simulink model "VTOLDynamics"  (R2024b)
settings: Solver=ode23t  StartTime=0.0  StopTime=10.0  FixedStep=0.001  RelTol=1e-3
undefined symbols (not defined in the file): const, contact, env, F, Flap_Activate, iniRoll, initPitch, iniYaw, Light, Limit, MIL, motorctrl, tiltIni, uavParam, uavParams, vIni, xGround, yGround, zGround
libraries: matrix_library x8, slpidlib x4, robotcorelib x4, aerolibasang x2, aerolibwind2 x2, sharedtransform x2, shared6dof x1, aerolibadyn x1, sharedutil x1, Uav_Electrical_lib x1, aerolibatmos2 x1
(part 2 of 3)

== system VTOLDynamics/Force and Moments/Propulsion/Rotor1 Drag Torque ==
  note: RPM_2_rad/s
  note: Drage Torque Calculate
      |
      | Vertical takeoff :
      |
      | Q = rho * A * (Omega*R)^2 * R * CQ, where the unit of Q is [N-m]
  note: Parameters
      | rho : air density
      | A : rotor blade area
      | Omega : motor speed (rad/s)
      | CQ: motor torque coefficient
      | R : rotor blade radius
  Actuator : Inport
  Gain1 : Gain  Gain=uavParams.aero.air_density*uavParams.geom.RotorArea*(uavParams.geom.PropDiameter/2)^3*uavParams.rotor.Cq
  Gain8 : Gain  Gain=2*pi/60
  Square : Math  Operator=square
  Unit Delay : UnitDelay  SampleTime=0.001  HasFrameUpgradeWarning=on
  Out1 : Outport
  wires:
  Gain8/1 -> Square/1
  Square/1 -> Gain1/1
  Actuator/1 -> Gain8/1
  Gain1/1 -> Unit Delay/1
  Unit Delay/1 -> Out1/1

== system VTOLDynamics/Force and Moments/Propulsion/Rotor2 Drag Torque ==
  note: RPM_2_rad/s
  note: Drage Torque Calculate
  Actuator : Inport
  Gain1 : Gain  Gain=uavParams.aero.air_density*uavParams.geom.RotorArea*(uavParams.geom.PropDiameter/2)^3*uavParams.rotor.Cq
  Gain8 : Gain  Gain=2*pi/60
  Square : Math  Operator=square
  Unit Delay : UnitDelay  SampleTime=0.001  HasFrameUpgradeWarning=on
  Out2 : Outport
  wires:
  Gain8/1 -> Square/1
  Square/1 -> Gain1/1
  Actuator/1 -> Gain8/1
  Gain1/1 -> Unit Delay/1
  Unit Delay/1 -> Out2/1

== system VTOLDynamics/Force and Moments/Propulsion/Rotor3 Drag Torque ==
  note: RPM_2_rad/s
  note: Drage Torque Calculate
  Actuator : Inport
  Gain1 : Gain  Gain=uavParams.aero.air_density*uavParams.geom.RotorArea*(uavParams.geom.PropDiameter/2)^3*uavParams.rotor.Cq
  Gain8 : Gain  Gain=2*pi/60
  Square : Math  Operator=square
  Unit Delay : UnitDelay  SampleTime=0.001  HasFrameUpgradeWarning=on
  Out2 : Outport
  wires:
  Gain8/1 -> Square/1
  Square/1 -> Gain1/1
  Actuator/1 -> Gain8/1
  Gain1/1 -> Unit Delay/1
  Unit Delay/1 -> Out2/1

== system VTOLDynamics/Force and Moments/Propulsion/Rotor4 Drag Torque ==
  note: RPM_2_rad/s
  note: Drage Torque Calculate
  Actuator : Inport
  Gain1 : Gain  Gain=uavParams.aero.air_density*uavParams.geom.RotorArea*(uavParams.geom.PropDiameter/2)^3*uavParams.rotor.Cq
  Gain8 : Gain  Gain=2*pi/60
  Square : Math  Operator=square
  Unit Delay : UnitDelay  SampleTime=0.001  HasFrameUpgradeWarning=on
  Out1 : Outport
  wires:
  Gain8/1 -> Square/1
  Square/1 -> Gain1/1
  Actuator/1 -> Gain8/1
  Gain1/1 -> Unit Delay/1
  Unit Delay/1 -> Out1/1

== system VTOLDynamics/Force and Moments/Propulsion/Tilt Servo Dynamics ==
  TiltA : Inport
  TiltB : Inport  Port=2
  Gain2 : Gain  Gain=pi/2
  Gain3 : Gain  Gain=pi/2
  IC : InitialCondition  Value=tiltIni
  IC1 : InitialCondition  Value=tiltIni
  Servo Dynamics : TransferFcn  Numerator=uavParams.tiltservo.tfnum  Denominator=uavParams.tiltservo.tfden
  Servo Dynamics1 : TransferFcn  Numerator=uavParams.tiltservo.tfnum  Denominator=uavParams.tiltservo.tfden
  Tilt1 : Outport
  Tilt2 : Outport  Port=2
  wires:
  Gain2/1 -> Servo Dynamics/1
  TiltB/1 -> Gain3/1
  Servo Dynamics/1 -> IC1/1
  Servo Dynamics1/1 -> IC/1
  IC/1 -> Tilt2/1  "Tilt2"
  IC1/1 -> Tilt1/1  "Tilt1"
  Gain3/1 -> Servo Dynamics1/1
  TiltA/1 -> Gain2/1

== system VTOLDynamics/Force and Moments/Weather Model/Simple Model ==
  note: #11, 25/07/04, MH, Fixed
      | Use International Standard Atmosphere model
      | to obtain the air density varying with altitude
  AirData : Inport
  Xe : Inport  Port=2
  Euler : Inport  Port=3
  Constant : Constant  Value=[ 0 0 0]
      settings: AttributesFormatString=%<Value>
  Constant1 : Constant  Commented=on  Value=const.rho0
  Gain : Gain  Gain=-1
  ISA Atmosphere Model : aerolibatmos2/ISA Atmosphere Model  useExtended=off  action=Warning  custom=off  viscosityOut=off  g=9.80665  gamma=1.4  R=287.0531  L=0.0065  h_trop=11000  h_strat=20000  rho0=1.225  P0=101325  T0=288.15  h0=0  S=110.4  Tref=273.15  muref=1.716e-5
  Selector : Selector  InputPortWidth=3  IndexOptions=Index vector (dialog)  Indices=[3]  OutputSizes=1
  Terminator{,1..4} (5 alike) : Terminator
  Wind_e : Outport  Unit=m/s  VectorParamsAs1DForOutWhenUnconnected=off
  " Rho" : Outport  Port=2  VectorParamsAs1DForOutWhenUnconnected=off
  wires:
  AirData/1 -> Terminator/1
  Constant/1 -> Wind_e/1
  Euler/1 -> Terminator1/1
  Xe/1 -> Selector/1
  Selector/1 -> Gain/1
  Gain/1 -> ISA Atmosphere Model/1
  ISA Atmosphere Model/1 -> Terminator2/1
  ISA Atmosphere Model/2 -> Terminator3/1
  ISA Atmosphere Model/3 -> Terminator4/1
  ISA Atmosphere Model/4 -> " Rho"/1

== system VTOLDynamics/Force and Moments/Weather Model/Weather Model ==
  note: 90 degree : East to West
      | 270 degree : West to East
      | 0 degree : North to South
      | 180 degree : South to North
  AirData : Inport
  Xe : Inport  Port=2
  Euler : Inport  Port=3
  Add : Sum  Inputs=2
  Bus Selector : BusSelector  OutputSignals=airspeed
  Constant1 : Constant  Value=uavParams.aero.air_density
  Dryden Wind Turbulence Model (Discrete (+q -r)) : aerolibwind2/Dryden Wind Turbulence Model  (Continuous (+q -r))  Commented=on  units=Metric (MKS)  spec=MIL-F-8785C  model=Discrete Dryden (+q -r)  W20=env.windBase/4  Wdeg=env.windDirTurb  TurbProb=10^-2 - Light  L_high=533.4  Wingspan=uavParam.geom.b  ts=0.005  Seed=[23341 23342 23343 23344]  T_on=on
  Gain : Gain  Gain=-1
      settings: AttributesFormatString=Z to Alt
  Get Z : Selector  InputPortWidth=3  IndexOptions=Index vector (dialog)  Indices=[3]  OutputSizes=[(-2)]
  Horizontal Wind Model : aerolibwind2/Horizontal Wind Model  units=Metric (MKS)  Vw_source=Internal  Vwind=Wind_Speed  W_source=Internal  Wdeg=90
  Reduce Z Wind1 : Gain  Gain=[1 1 0.1]
      settings: AttributesFormatString=%<Gain>
  Rotate to E Frame : Product  Multiplication=Matrix(*)
  Rotation Angles to Direction Cosine Matrix : sharedtransform/Rotation Angles to Direction Cosine Matrix  rotationOrder=ZYX  aMode=aMode
  Selector : Selector  InputPortWidth=3  IndexOptions=Index vector (dialog)  Indices=[3 2 1]  OutputSizes=1
  Terminator : Terminator
  Terminator1 : Terminator
  Transfer Fcn : TransferFcn  Denominator=[.01 1]
  Transfer Fcn1 : TransferFcn  Denominator=[.01 1]
  Transpose : Math  Operator=transpose  SignedPower=on
  Wind_e : Outport  Unit=m/s  VectorParamsAs1DForOutWhenUnconnected=off
  Rho : Outport  Port=2  VectorParamsAs1DForOutWhenUnconnected=off
  wires:
  Bus Selector/1 -> Transfer Fcn1/1  "<airspeed>"
  AirData/1 -> Bus Selector/1
  Transfer Fcn/1 -> Gain/1
  Dryden Wind Turbulence Model (Discrete (+q -r))/2 -> Terminator/1
  Dryden Wind Turbulence Model (Discrete (+q -r))/1 -> Terminator1/1
  Rotate to E Frame/1 -> Wind_e/1
  Transpose/1 -> Rotate to E Frame/1
  Transfer Fcn1/1 -> Dryden Wind Turbulence Model (Discrete (+q -r))/2
  Add/1 -> Rotate to E Frame/2
  Rotation Angles to Direction Cosine Matrix/1 -> Horizontal Wind Model/1, Dryden Wind Turbulence Model (Discrete (+q -r))/3, Transpose/1  "RECEF2B"
  Get Z/1 -> Transfer Fcn/1
  Xe/1 -> Get Z/1
  Gain/1 -> Dryden Wind Turbulence Model (Discrete (+q -r))/1
  Constant1/1 -> Rho/1
  Selector/1 -> Rotation Angles to Direction Cosine Matrix/1
  Euler/1 -> Selector/1
  Horizontal Wind Model/1 -> Add/2

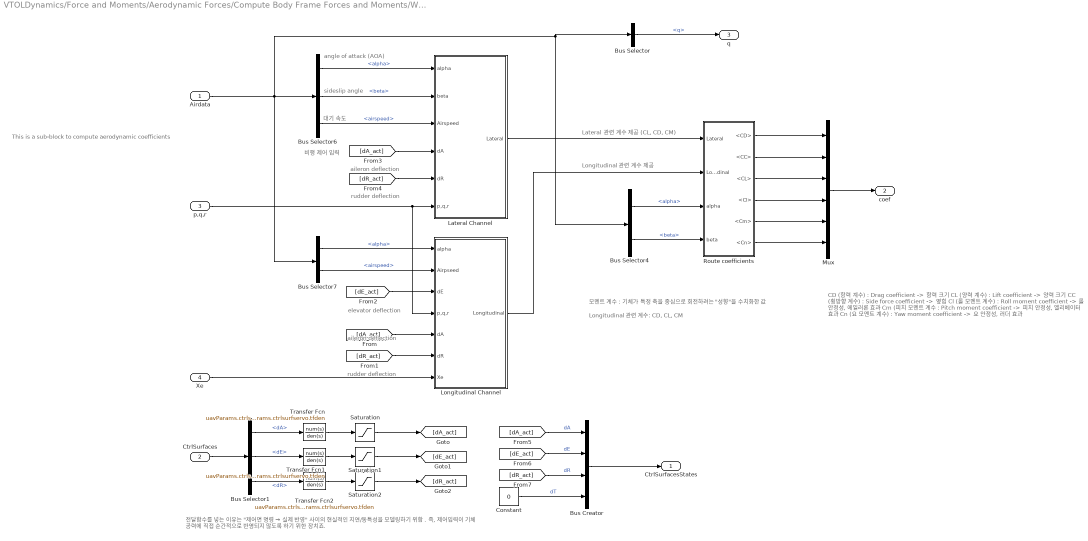
== system VTOLDynamics/Force and Moments/Aerodynamic Forces/Compute Body Frame Forces and Moments/Wind frame F& M ==
  note: CD (항력 계수) : Drag coefficient -> 항력 크기
      | CL (양력 계수) : Lift coefficient -> 양력 크기
      | CC (횡방향 계수) : Side force coefficient -> 옆힘
      | Cl (롤 모멘트 계수) : Roll moment coefficient -> 롤 안정성, 에일러론 효과
      | Cm (피치 모멘트 계수 : Pitch moment coefficient -> 피치 안정성, 엘리베이터 효과
      | Cn (요 모멘트 계수) : Yaw moment coefficient -> 요 안정성, 러더 효과
  note: 전달함수를 넣는 이유는 "제어면 명령 → 실제 반영" 사이의 현실적인 지연/동특성을 모델링하기 위함 .
      | 즉, 제어입력이 기체 공력에 직접 순간적으로 반영되지 않도록 하기 위한 장치죠.
  note: aileron deflection
  note: This is a sub-block to compute aerodynamic coefficients
  note: angle of attack (AOA)
  note: sideslip angle
  note: rudder deflection
  note: elevator deflection
  note: 비행 제어 입력
  note: Lateral 관련 계수 제공 (CL, CD, CM)
  note: Longitudinal 관련 계수 제공
  note: rudder deflection
  note: aileron deflection
  note: 모멘트 계수 : 기체가 특정 축을 중심으로 회전하려는 "성향"을 수치화한 값
  note: 대기 속도
  note: Longitudinal 관련 계수: CD, CL, CM
  Airdata : Inport
  CtrlSurfaces : Inport  Port=2
  p,q,r : Inport  Port=3
  Xe : Inport  Port=4
  Bus Creator : BusCreator  Inputs=4  OutDataTypeStr=Bus: FixedWingCtrlBus
  Bus Selector : BusSelector  OutputSignals=q
  Bus Selector1 : BusSelector  OutputSignals=dA,dE,dR
  Bus Selector4 : BusSelector  OutputSignals=alpha,beta
  Bus Selector6 : BusSelector  OutputSignals=alpha,beta,airspeed
  Bus Selector7 : BusSelector  OutputSignals=alpha,airspeed
  Constant : Constant  Value=0
  Lateral Channel : Subsystem
  Longitudinal Channel : Subsystem
  Mux : Mux  Inputs=6
  Route coefficients : Subsystem
  Saturation : Saturate  UpperLimit=uavParams.maxAileron  LowerLimit=uavParams.minAileron
  Saturation1 : Saturate  UpperLimit=uavParams.maxElevator  LowerLimit=uavParams.minElevator
  Saturation2 : Saturate  UpperLimit=uavParams.maxRudder  LowerLimit=uavParams.minRudder
  Transfer Fcn : TransferFcn  Numerator=uavParams.ctrlsurfservo.tfnum  Denominator=uavParams.ctrlsurfservo.tfden
  Transfer Fcn1 : TransferFcn  Numerator=uavParams.ctrlsurfservo.tfnum  Denominator=uavParams.ctrlsurfservo.tfden
  Transfer Fcn2 : TransferFcn  Numerator=uavParams.ctrlsurfservo.tfnum  Denominator=uavParams.ctrlsurfservo.tfden
  CtrlSurfacesStates : Outport  VectorParamsAs1DForOutWhenUnconnected=off
  coef : Outport  Port=2  PortDimensions=6  VectorParamsAs1DForOutWhenUnconnected=off
  q : Outport  Port=3
  wires:
  Bus Selector7/2 -> Longitudinal Channel/2(Airpseed)  "<airspeed>"
  Bus Selector7/1 -> Longitudinal Channel/1(alpha)  "<alpha>"
  Bus Selector6/3 -> Lateral Channel/3(Airspeed)  "<airspeed>"
  Bus Selector6/2 -> Lateral Channel/2(beta)  "<beta>"
  Airdata/1 -> Bus Selector/1, Bus Selector4/1, Bus Selector7/1, Bus Selector6/1
  p,q,r/1 -> Longitudinal Channel/4(p,q,r), Lateral Channel/6(p,q,r)
  Mux/1 -> coef/1
  Longitudinal Channel/1(Longitudinal) -> Route coefficients/2(Longitudinal)
  Route coefficients/1(<CD>) -> Mux/1
  Route coefficients/2(<CC>) -> Mux/2
  Route coefficients/3(<CL>) -> Mux/3
  Route coefficients/4(<Cl>) -> Mux/4
  Route coefficients/5(<Cm>) -> Mux/5
  Route coefficients/6(<Cn>) -> Mux/6
  Bus Selector/1 -> q/1  "<q>"
  Lateral Channel/1(Lateral) -> Route coefficients/1(Lateral)
  Bus Selector4/1 -> Route coefficients/3(alpha)  "<alpha>"
  Bus Selector4/2 -> Route coefficients/4(beta)  "<beta>"
  Bus Selector6/1 -> Lateral Channel/1(alpha)  "<alpha>"
  Transfer Fcn/1 -> Saturation/1
  Transfer Fcn1/1 -> Saturation1/1
  Transfer Fcn2/1 -> Saturation2/1
  [dA_act] -> Longitudinal Channel/5(dA)
  [dR_act] -> Longitudinal Channel/6(dR)
  [dE_act] -> Longitudinal Channel/3(dE)
  [dA_act] -> Lateral Channel/4(dA)
  [dR_act] -> Lateral Channel/5(dR)
  CtrlSurfaces/1 -> Bus Selector1/1
  Bus Creator/1 -> CtrlSurfacesStates/1
  [dA_act] -> Bus Creator/1  "dA"
  [dE_act] -> Bus Creator/2  "dE"
  [dR_act] -> Bus Creator/3  "dR"
  Constant/1 -> Bus Creator/4  "dT"
  Bus Selector1/1 -> Transfer Fcn/1  "<dA>"
  Bus Selector1/2 -> Transfer Fcn1/1  "<dE>"
  Bus Selector1/3 -> Transfer Fcn2/1  "<dR>"
  Saturation/1 -> [dA_act]
  Saturation2/1 -> [dR_act]
  Saturation1/1 -> [dE_act]
  Xe/1 -> Longitudinal Channel/7(Xe)

== system VTOLDynamics/Force and Moments/Aerodynamic Forces/Compute Body Frame Forces and Moments/Wind frame F& M_original ==
  Airdata : Inport
  CtrlSurfaces : Inport  Port=2
  p,q,r : Inport  Port=3
  Bus Selector : BusSelector  OutputSignals=q
  Bus Selector1 : BusSelector  OutputSignals=dA,dR
  Bus Selector2 : BusSelector  OutputSignals=dE,dA,dR
  Bus Selector6 : BusSelector  OutputSignals=beta,airspeed
  Bus Selector7 : BusSelector  OutputSignals=alpha,airspeed
  Lateral Channel : Subsystem
  Longitudinal Channel : Subsystem
  Mux : Mux  Inputs=6
  Route coefficients : Subsystem
  coef : Outport  PortDimensions=6  VectorParamsAs1DForOutWhenUnconnected=off
  q : Outport  Port=2
  wires:
  Bus Selector7/2 -> Longitudinal Channel/2(Airpseed)  "<airspeed>"
  Bus Selector7/1 -> Longitudinal Channel/1(alpha)  "<alpha>"
  Bus Selector6/2 -> Lateral Channel/2(Airspeed)  "<airspeed>"
  Bus Selector6/1 -> Lateral Channel/1(beta)  "<beta>"
  Airdata/1 -> Bus Selector/1, Bus Selector6/1, Bus Selector7/1
  Bus Selector2/1 -> Longitudinal Channel/3(dE)  "<dE>"
  Bus Selector1/2 -> Lateral Channel/4(dR)  "<dR>"
  Bus Selector1/1 -> Lateral Channel/3(dA)  "<dA>"
  CtrlSurfaces/1 -> Bus Selector1/1, Bus Selector2/1
  p,q,r/1 -> Lateral Channel/5(p,q,r), Longitudinal Channel/4(p,q,r)
  Bus Selector2/2 -> Longitudinal Channel/5(dA)  "<dA>"
  Bus Selector2/3 -> Longitudinal Channel/6(dR)  "<dR>"
  Mux/1 -> coef/1
  Lateral Channel/1(Lateral) -> Route coefficients/1(Lateral)
  Longitudinal Channel/1(Longitudinal) -> Route coefficients/2(Longitudinal)
  Route coefficients/1(<CD>) -> Mux/1
  Route coefficients/2(<CY>) -> Mux/2
  Route coefficients/3(<CL>) -> Mux/3
  Route coefficients/4(<Cl>) -> Mux/4
  Route coefficients/5(<Cm>) -> Mux/5
  Route coefficients/6(<Cn>) -> Mux/6
  Bus Selector/1 -> q/1  "<q>"

== system VTOLDynamics/Force and Moments/Ground Model/Friction Force/Soft Coulomb Friction ==
  note: Pennestrì, E., Rossi, V., Salvini, P. et al. Review and comparison of dry friction force models. Nonlinear Dyn 83, 1785–1801 (2016). https://doi.org/10.1007/s11071-015-2485-3
  V : Inport
  Tanh : Trigonometry  Operator=tanh
  friction coefficient : Gain  Gain=contact.rollingFriction*1.2
  vd : Gain  Gain=1/contact.vd
  Out1 : Outport
  wires:
  V/1 -> vd/1
  vd/1 -> Tanh/1
  Tanh/1 -> friction coefficient/1
  friction coefficient/1 -> Out1/1

== system VTOLDynamics/Force and Moments/Propulsion/Rotor Assembly 1/Adjust Force to Body Frame ==
  Fmotor : Inport
  Tilt : Inport  Port=2
  TurnDirection : Inport  Port=3
  Constant : Constant
  Constant1 : Constant
  Constant2 : Constant  Value=0
  Constant3 : Constant  Value=0
  Coordinate Transformation Conversion : robotcorelib/Coordinate Transformation Conversion  InputRepresentation=Euler Angles  InputEulerSequence=ZYX  ShowTrVecInputPort=on  OutputRepresentation=Rotation Matrix  OutputEulerSequence=ZYX  ShowTrVecOutputPort=on  SimulateUsing=Code generation
      settings: LibrarySourceBlock=uavutilslib/Coordinate Transformation Conversion
  Gain2 : Gain  Gain=-1
  Mux : Mux  Inputs=3
  Mux1 : Mux  Inputs=3
  Product : Product
  Product2 : Product  Multiplication=Matrix(*)
  Fbody : Outport
  wires:
  Constant1/1 -> Mux/3
  Constant/1 -> Mux/1
  Constant3/1 -> Mux1/3
  Constant2/1 -> Mux1/1
  Product2/1 -> Fbody/1
  Coordinate Transformation Conversion/1 -> Product2/1
  Mux/1 -> Product/2
  Product/1 -> Product2/2
  Gain2/1 -> Mux1/2
  TurnDirection/1 -> Mux/2
  Mux1/1 -> Coordinate Transformation Conversion/1
  Tilt/1 -> Gain2/1
  Fmotor/1 -> Product/1

== system VTOLDynamics/Force and Moments/Propulsion/Rotor Assembly 1/Compute motor base velocity ==
  Vb : Inport
  a : Inport  Port=2
  b : Inport  Port=3
  Add : Sum
  Cross Product : matrix_library/Cross Product
  Reshape : Reshape  OutputDimensionality=Column vector (2-D)
  Vmotor : Outport
  wires:
  b/1 -> Cross Product/2
  a/1 -> Cross Product/1
  Vb/1 -> Reshape/1
  Cross Product/1 -> Add/2
  Add/1 -> Vmotor/1
  Reshape/1 -> Add/1

== system VTOLDynamics/Force and Moments/Propulsion/Rotor Assembly 2/Adjust Force to Body Frame ==
  Fmotor : Inport
  Tilt : Inport  Port=2
  TurnDirection : Inport  Port=3
  Constant : Constant
  Constant1 : Constant
  Constant2 : Constant  Value=0
  Constant3 : Constant  Value=0
  Coordinate Transformation Conversion : robotcorelib/Coordinate Transformation Conversion  InputRepresentation=Euler Angles  InputEulerSequence=ZYX  ShowTrVecInputPort=on  OutputRepresentation=Rotation Matrix  OutputEulerSequence=ZYX  ShowTrVecOutputPort=on  SimulateUsing=Code generation
      settings: LibrarySourceBlock=uavutilslib/Coordinate Transformation Conversion
  Gain2 : Gain  Gain=-1
  Mux : Mux  Inputs=3
  Mux1 : Mux  Inputs=3
  Product : Product
  Product2 : Product  Multiplication=Matrix(*)
  Fbody : Outport
  wires:
  Constant1/1 -> Mux/3
  Constant/1 -> Mux/1
  Constant3/1 -> Mux1/3
  Constant2/1 -> Mux1/1
  Product2/1 -> Fbody/1
  Coordinate Transformation Conversion/1 -> Product2/1
  Mux/1 -> Product/2
  Product/1 -> Product2/2
  Gain2/1 -> Mux1/2
  TurnDirection/1 -> Mux/2
  Mux1/1 -> Coordinate Transformation Conversion/1
  Tilt/1 -> Gain2/1
  Fmotor/1 -> Product/1

== system VTOLDynamics/Force and Moments/Propulsion/Rotor Assembly 2/Compute motor base velocity ==
  Vb : Inport
  a : Inport  Port=2
  b : Inport  Port=3
  Add : Sum
  Cross Product : matrix_library/Cross Product
  Reshape : Reshape  OutputDimensionality=Column vector (2-D)
  Vmotor : Outport
  wires:
  b/1 -> Cross Product/2
  a/1 -> Cross Product/1
  Vb/1 -> Reshape/1
  Cross Product/1 -> Add/2
  Add/1 -> Vmotor/1
  Reshape/1 -> Add/1

== system VTOLDynamics/Force and Moments/Propulsion/Rotor Assembly 3/Adjust Force to Body Frame ==
  Fmotor : Inport
  Tilt : Inport  Port=2
  TurnDirection : Inport  Port=3
  Constant : Constant
  Constant1 : Constant
  Constant2 : Constant  Value=0
  Constant3 : Constant  Value=0
  Coordinate Transformation Conversion : robotcorelib/Coordinate Transformation Conversion  InputRepresentation=Euler Angles  InputEulerSequence=ZYX  ShowTrVecInputPort=on  OutputRepresentation=Rotation Matrix  OutputEulerSequence=ZYX  ShowTrVecOutputPort=on  SimulateUsing=Code generation
      settings: LibrarySourceBlock=uavutilslib/Coordinate Transformation Conversion
  Gain2 : Gain  Gain=-1
  Mux : Mux  Inputs=3
  Mux1 : Mux  Inputs=3
  Product : Product
  Product2 : Product  Multiplication=Matrix(*)
  Fbody : Outport
  wires:
  Constant1/1 -> Mux/3
  Constant/1 -> Mux/1
  Constant3/1 -> Mux1/3
  Constant2/1 -> Mux1/1
  Product2/1 -> Fbody/1
  Coordinate Transformation Conversion/1 -> Product2/1
  Mux/1 -> Product/2
  Product/1 -> Product2/2
  Gain2/1 -> Mux1/2
  TurnDirection/1 -> Mux/2
  Mux1/1 -> Coordinate Transformation Conversion/1
  Tilt/1 -> Gain2/1
  Fmotor/1 -> Product/1

== system VTOLDynamics/Force and Moments/Propulsion/Rotor Assembly 3/Compute motor base velocity ==
  Vb : Inport
  a : Inport  Port=2
  b : Inport  Port=3
  Add : Sum
  Cross Product : matrix_library/Cross Product
  Reshape : Reshape  OutputDimensionality=Column vector (2-D)
  Vmotor : Outport
  wires:
  b/1 -> Cross Product/2
  a/1 -> Cross Product/1
  Vb/1 -> Reshape/1
  Cross Product/1 -> Add/2
  Add/1 -> Vmotor/1
  Reshape/1 -> Add/1

== system VTOLDynamics/Force and Moments/Propulsion/Rotor Assembly 4/Adjust Force to Body Frame ==
  Fmotor : Inport
  Tilt : Inport  Port=2
  TurnDirection : Inport  Port=3
  Constant : Constant
  Constant1 : Constant
  Constant2 : Constant  Value=0
  Constant3 : Constant  Value=0
  Coordinate Transformation Conversion : robotcorelib/Coordinate Transformation Conversion  InputRepresentation=Euler Angles  InputEulerSequence=ZYX  ShowTrVecInputPort=on  OutputRepresentation=Rotation Matrix  OutputEulerSequence=ZYX  ShowTrVecOutputPort=on  SimulateUsing=Code generation
      settings: LibrarySourceBlock=uavutilslib/Coordinate Transformation Conversion
  Gain2 : Gain  Gain=-1
  Mux : Mux  Inputs=3
  Mux1 : Mux  Inputs=3
  Product : Product
  Product2 : Product  Multiplication=Matrix(*)
  Fbody : Outport
  wires:
  Constant1/1 -> Mux/3
  Constant/1 -> Mux/1
  Constant3/1 -> Mux1/3
  Constant2/1 -> Mux1/1
  Product2/1 -> Fbody/1
  Coordinate Transformation Conversion/1 -> Product2/1
  Mux/1 -> Product/2
  Product/1 -> Product2/2
  Gain2/1 -> Mux1/2
  TurnDirection/1 -> Mux/2
  Mux1/1 -> Coordinate Transformation Conversion/1
  Tilt/1 -> Gain2/1
  Fmotor/1 -> Product/1

== system VTOLDynamics/Force and Moments/Propulsion/Rotor Assembly 4/Compute motor base velocity ==
  Vb : Inport
  a : Inport  Port=2
  b : Inport  Port=3
  Add : Sum
  Cross Product : matrix_library/Cross Product
  Reshape : Reshape  OutputDimensionality=Column vector (2-D)
  Vmotor : Outport
  wires:
  b/1 -> Cross Product/2
  a/1 -> Cross Product/1
  Vb/1 -> Reshape/1
  Cross Product/1 -> Add/2
  Add/1 -> Vmotor/1
  Reshape/1 -> Add/1

== system VTOLDynamics/Force and Moments/Aerodynamic Forces/Compute Body Frame Forces and Moments/Wind frame F& M/Lateral Channel ==
  alpha : Inport
  beta : Inport  Port=2
  Airspeed : Inport  Port=3
  dA : Inport  Port=4
  dR : Inport  Port=5
  p,q,r : Inport  Port=6
  Bus Creator : BusCreator  Inputs=3
  CY : Subsystem
  Cl : Subsystem
  Cn : Subsystem
  Lateral : Outport  VectorParamsAs1DForOutWhenUnconnected=off
  wires:
  p,q,r/1 -> CY/4(p,q,r), Cl/5(p,q,r), Cn/5(p,q,r)
  Airspeed/1 -> CY/5(Airspeed), Cl/6(Airspeed), Cn/6(Airspeed)
  dR/1 -> CY/3(dR), Cl/4(dR), Cn/4(dR)
  dA/1 -> Cn/3(dA), Cl/3(dA)
  beta/1 -> CY/2(beta), Cn/2(beta), Cl/2(beta)
  Bus Creator/1 -> Lateral/1
  CY/1(CS) -> Bus Creator/1  "CS"
  alpha/1 -> Cl/1(alpha), Cn/1(alpha), CY/1(alpha)
  Cl/1(Cl) -> Bus Creator/2  "Cl"
  Cn/1(Cn) -> Bus Creator/3  "Cn"

== system VTOLDynamics/Force and Moments/Aerodynamic Forces/Compute Body Frame Forces and Moments/Wind frame F& M/Longitudinal Channel ==
  alpha : Inport
  Airpseed : Inport  Port=2
  dE : Inport  Port=3
  p,q,r : Inport  Port=4
  dA : Inport  Port=5
  dR : Inport  Port=6
  Xe : Inport  Port=7
  Bus Creator : BusCreator  Inputs=3
  CD : Subsystem
  CL : Subsystem
  Cm : Subsystem
  Saturation : Saturate  UpperLimit=max(uavParams.aero.alpha_lon)  LowerLimit=min(uavParams.aero.alpha_lon)  ZeroCross=off
  Selector : Selector  InputPortWidth=3  IndexOptions=Index vector (dialog)  Indices=[1]  OutputSizes=1
  Transfer Fcn : TransferFcn  Numerator=uavParams.aero.CLadot_tfnum  Denominator=uavParams.aero.CLadot_tfden
  Longitudinal : Outport  VectorParamsAs1DForOutWhenUnconnected=off
  wires:
  Airpseed/1 -> Cm/4(Airspeed), CL/5(Airspeed)
  p,q,r/1 -> CL/4(p,q,r), Cm/3(p,q,r)
  Bus Creator/1 -> Longitudinal/1
  dE/1 -> CL/3(dE), Cm/2(dE), CD/4(dE)
  CD/1(CD) -> Bus Creator/1  "CD"
  alpha/1 -> Saturation/1
  dR/1 -> CD/3(dR)
  dA/1 -> CD/2(dA), CL/6(dA)
  Saturation/1 -> CD/1(alpha), Cm/1(alpha), CL/1(alpha), Transfer Fcn/1
  Cm/1(Cm) -> Bus Creator/3  "Cm"
  CL/1(CL) -> Bus Creator/2  "CL"
  Transfer Fcn/1 -> CL/2(alpha_dot)
  Xe/1 -> Selector/1
  Selector/1 -> Cm/5(Xe), CL/7(Xe), CD/5(Xe)

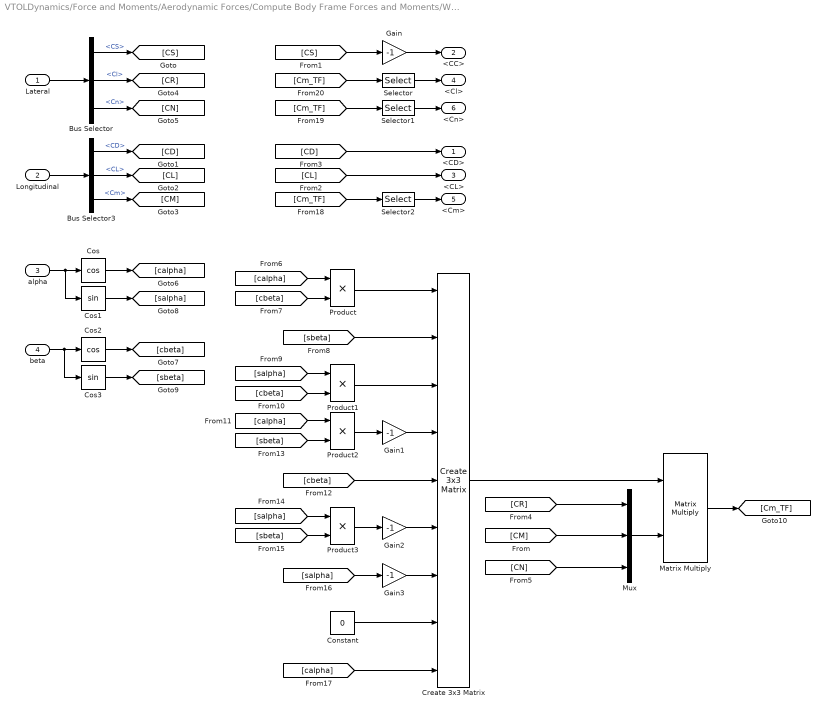
== system VTOLDynamics/Force and Moments/Aerodynamic Forces/Compute Body Frame Forces and Moments/Wind frame F& M/Route coefficients ==
  Lateral : Inport
  Longitudinal : Inport  Port=2
  alpha : Inport  Port=3
  beta : Inport  Port=4
  Bus Selector : BusSelector  OutputSignals=CS,Cl,Cn
  Bus Selector3 : BusSelector  OutputSignals=CD,CL,Cm
  Constant : Constant  Value=0
  Cos : Trigonometry  Operator=cos
  Cos1 : Trigonometry
  Cos2 : Trigonometry  Operator=cos
  Cos3 : Trigonometry
  Create 3x3 Matrix : sharedutil/Create 3x3 Matrix  aMode=aMode
      settings: LibrarySourceBlock=aerolibutil/Create 3x3 Matrix
  Gain{,1..3} (4 alike) : Gain  Gain=-1
  Matrix Multiply : Product  Multiplication=Matrix(*)
  Mux : Mux  Inputs=3
  Product{,1..3} (4 alike) : Product
  Selector : Selector  InputPortWidth=3  IndexOptions=Index vector (dialog)  Indices=[1]  OutputSizes=1
  Selector1 : Selector  InputPortWidth=3  IndexOptions=Index vector (dialog)  Indices=[3]  OutputSizes=1
  Selector2 : Selector  InputPortWidth=3  IndexOptions=Index vector (dialog)  Indices=[2]  OutputSizes=1
  <CD> : Outport
  <CC> : Outport  Port=2
  <CL> : Outport  Port=3
  <Cl> : Outport  Port=4
  <Cm> : Outport  Port=5
  <Cn> : Outport  Port=6
  wires:
  Lateral/1 -> Bus Selector/1
  Longitudinal/1 -> Bus Selector3/1
  Bus Selector/1 -> [CS]  "<CS>"
  Bus Selector3/1 -> [CD]  "<CD>"
  Bus Selector3/2 -> [CL]  "<CL>"
  [CL] -> <CL>/1
  [CD] -> <CD>/1
  Bus Selector3/3 -> [CM]  "<Cm>"
  Bus Selector/2 -> [CR]  "<Cl>"
  Bus Selector/3 -> [CN]  "<Cn>"
  Cos/1 -> [calpha]
  alpha/1 -> Cos1/1, Cos/1
  Cos1/1 -> [salpha]
  Cos2/1 -> [cbeta]
  Cos3/1 -> [sbeta]
  beta/1 -> Cos3/1, Cos2/1
  [calpha] -> Product/1
  [cbeta] -> Product/2
  Product/1 -> Create 3x3 Matrix/1
  [sbeta] -> Create 3x3 Matrix/2
  Product1/1 -> Create 3x3 Matrix/3
  [salpha] -> Product1/1
  [cbeta] -> Product1/2
  [calpha] -> Product2/1
  Product2/1 -> Gain1/1
  [sbeta] -> Product2/2
  Gain1/1 -> Create 3x3 Matrix/4
  [cbeta] -> Create 3x3 Matrix/5
  Product3/1 -> Gain2/1
  [salpha] -> Product3/1
  [sbeta] -> Product3/2
  Gain2/1 -> Create 3x3 Matrix/6
  Gain3/1 -> Create 3x3 Matrix/7
  [salpha] -> Gain3/1
  Constant/1 -> Create 3x3 Matrix/8
  [calpha] -> Create 3x3 Matrix/9
  Create 3x3 Matrix/1 -> Matrix Multiply/1
  Mux/1 -> Matrix Multiply/2
  [CM] -> Mux/2
  Matrix Multiply/1 -> [Cm_TF]
  [Cm_TF] -> Selector/1
  [Cm_TF] -> Selector1/1
  [Cm_TF] -> Selector2/1
  [CR] -> Mux/1
  [CN] -> Mux/3
  Gain/1 -> <CC>/1
  [CS] -> Gain/1
  Selector2/1 -> <Cm>/1
  Selector/1 -> <Cl>/1
  Selector1/1 -> <Cn>/1

== system VTOLDynamics/Force and Moments/Aerodynamic Forces/Compute Body Frame Forces and Moments/Wind frame F& M_original/Lateral Channel ==
  beta : Inport
  Airspeed : Inport  Port=2
  dA : Inport  Port=3
  dR : Inport  Port=4
  p,q,r : Inport  Port=5
  Bus Creator : BusCreator  Inputs=3
  CY : Subsystem
  Cl : Subsystem
  Cn : Subsystem
  Lateral : Outport  VectorParamsAs1DForOutWhenUnconnected=off
  wires:
  Cl/1(Cl) -> Bus Creator/2  "Cl"
  p,q,r/1 -> CY/3(p,q,r), Cn/4(p,q,r), Cl/4(p,q,r)
  Airspeed/1 -> CY/4(Airspeed), Cn/5(Airspeed), Cl/5(Airspeed)
  dR/1 -> CY/2(dR), Cl/3(dR), Cn/3(dR)
  dA/1 -> Cl/2(dA), Cn/2(dA)
  beta/1 -> CY/1(beta), Cl/1(beta), Cn/1(beta)
  Cn/1(Cn) -> Bus Creator/3  "Cn"
  CY/1(CY) -> Bus Creator/1  "CY"
  Bus Creator/1 -> Lateral/1

== system VTOLDynamics/Force and Moments/Aerodynamic Forces/Compute Body Frame Forces and Moments/Wind frame F& M_original/Longitudinal Channel ==
  alpha : Inport
  Airpseed : Inport  Port=2
  dE : Inport  Port=3
  p,q,r : Inport  Port=4
  dA : Inport  Port=5
  dR : Inport  Port=6
  Bus Creator : BusCreator  Inputs=3
  CD : Subsystem
  CL : Subsystem
  Cm : Subsystem
  Saturation : Saturate  UpperLimit=14*pi/180  LowerLimit=-14*pi/180  LinearizeAsGain=off  ZeroCross=off
  Transfer Fcn : TransferFcn  Numerator=[1 0]  Denominator=[0.1 1]
  Y-down : Gain  SaturateOnIntegerOverflow=on  OutDataTypeStr=Inherit: Same as input  ParamDataTypeStr=Inherit: Same as input
      settings: AttributesFormatString=%<Gain>
  Longitudinal : Outport  VectorParamsAs1DForOutWhenUnconnected=off
  wires:
  Transfer Fcn/1 -> CL/2(alpha_dot)
  Airpseed/1 -> Cm/4(Airspeed), CL/5(Airspeed)
  p,q,r/1 -> Cm/3(p,q,r), CL/4(p,q,r)
  Bus Creator/1 -> Longitudinal/1
  Cm/1(Cm) -> Bus Creator/3  "Cm"
  CL/1(CL) -> CD/1(CL), Y-down/1
  dE/1 -> Cm/2(De), CD/4(dE), CL/3(dE)
  Y-down/1 -> Bus Creator/2  "CL"
  CD/1(CD) -> Bus Creator/1  "CD"
  alpha/1 -> Saturation/1
  dR/1 -> CD/3(dR)
  dA/1 -> CD/2(dA), CL/6(dA)
  Saturation/1 -> Transfer Fcn/1, Cm/1(alpha), CL/1(alpha)

== system VTOLDynamics/Force and Moments/Aerodynamic Forces/Compute Body Frame Forces and Moments/Wind frame F& M_original/Route coefficients ==
  Lateral : Inport
  Longitudinal : Inport  Port=2
  Bus Selector : BusSelector  OutputSignals=CY,Cl,Cn
  Bus Selector3 : BusSelector  OutputSignals=CD,CL,Cm
  <CD> : Outport
  <CY> : Outport  Port=2
  <CL> : Outport  Port=3
  <Cl> : Outport  Port=4
  <Cm> : Outport  Port=5
  <Cn> : Outport  Port=6
  wires:
  Bus Selector3/2 -> <CL>/1  "<CL>"
  Bus Selector/3 -> <Cn>/1  "<Cn>"
  Bus Selector/2 -> <Cl>/1  "<Cl>"
  Lateral/1 -> Bus Selector/1
  Bus Selector3/3 -> <Cm>/1  "<Cm>"
  Bus Selector3/1 -> <CD>/1  "<CD>"
  Longitudinal/1 -> Bus Selector3/1
  Bus Selector/1 -> <CY>/1  "<CY>"

== system VTOLDynamics/Force and Moments/Aerodynamic Forces/Compute Body Frame Forces and Moments/Wind frame F& M/Lateral Channel/CY ==
  alpha : Inport
  beta : Inport  Port=2
  dR : Inport  Port=3
  p,q,r : Inport  Port=4
  Airspeed : Inport  Port=5
  1-D Lookup Table : Lookup_n-D  BreakpointsForDimension1=uavParams.aero.alpha_latdir  BreakpointsForDimension2=uavParams.aero.beta_latdir  Table=uavParams.aero.CS  ExtrapMethod=Clip  UseLastTableValue=on  InternalRulePriority=Speed  RndMeth=Simplest
      settings: InputPortMap=u0,u1
  Abs : Abs  Commented=on  SaturateOnIntegerOverflow=off
  CYDr : Constant  Value=uavParams.aero.CYDr
      settings: AttributesFormatString=%<Value>
  CYb : Constant  Commented=on  Value=uavParam.aero.CYb
      settings: AttributesFormatString=%<Value>
  Product : Product  Commented=on  SaturateOnIntegerOverflow=on  OutDataTypeStr=Inherit: Same as first input
  Product1 : Product  SaturateOnIntegerOverflow=on  OutDataTypeStr=Inherit: Same as first input
  Product2 : Product  Commented=on
  Sign : Signum  Commented=on
  Sum2 : Sum  Inputs=++++  SaturateOnIntegerOverflow=on
  roll factors : Subsystem
  CS : Outport  VectorParamsAs1DForOutWhenUnconnected=off
  wires:
  dR/1 -> Product1/2
  CYDr/1 -> Product1/1
  CYb/1 -> Product/1
  Airspeed/1 -> roll factors/2(Airspeed)
  p,q,r/1 -> roll factors/1(p,q,r)
  Sum2/1 -> CS/1
  beta/1 -> 1-D Lookup Table/2
  1-D Lookup Table/1 -> Sum2/1
  alpha/1 -> 1-D Lookup Table/1
  Sign/1 -> Product2/2
  Product1/1 -> Sum2/2
  roll factors/1(CSp) -> Sum2/3
  roll factors/2(CSr) -> Sum2/4

== system VTOLDynamics/Force and Moments/Aerodynamic Forces/Compute Body Frame Forces and Moments/Wind frame F& M/Lateral Channel/Cl ==
  alpha : Inport
  beta : Inport  Port=2
  dA : Inport  Port=3
  dR : Inport  Port=4
  p,q,r : Inport  Port=5
  Airspeed : Inport  Port=6
  1-D Lookup Table : Lookup_n-D  BreakpointsForDimension1=uavParams.aero.alpha_latdir  BreakpointsForDimension2=uavParams.aero.beta_latdir  Table=uavParams.aero.CR  InternalRulePriority=Speed  RndMeth=Simplest
      settings: InputPortMap=u0,u1
  Abs : Abs  Commented=on  SaturateOnIntegerOverflow=off
  ClDa : Constant  Value=uavParams.aero.ClDa
      settings: AttributesFormatString=%<Value>
  ClDr : Constant  Value=uavParams.aero.ClDr
      settings: AttributesFormatString=%<Value>
  Clb : Constant  Commented=on  Value=uavParam.aero.Clb
      settings: AttributesFormatString=%<Value>
  Product1 : Product  SaturateOnIntegerOverflow=on  OutDataTypeStr=Inherit: Same as first input
  Product2 : Product  Commented=on
  Product5 : Product  SaturateOnIntegerOverflow=on  OutDataTypeStr=Inherit: Same as first input
  Sign : Signum  Commented=on
  Sum : Sum  Inputs=+++++  SaturateOnIntegerOverflow=on
  roll factors : Subsystem
  Cl : Outport  VectorParamsAs1DForOutWhenUnconnected=off
  wires:
  roll factors/1(Clp) -> Sum/4
  Product5/1 -> Sum/2  "CldA"
  Airspeed/1 -> roll factors/2(Airspeed)
  p,q,r/1 -> roll factors/1(p,q,r)
  roll factors/2(Clr) -> Sum/5
  Product1/1 -> Sum/3  "Cldr"
  Sum/1 -> Cl/1
  dR/1 -> Product1/2
  ClDr/1 -> Product1/1
  dA/1 -> Product5/2
  ClDa/1 -> Product5/1
  Clb/1 -> ?
  beta/1 -> 1-D Lookup Table/2
  Sign/1 -> Product2/2
  alpha/1 -> 1-D Lookup Table/1
  1-D Lookup Table/1 -> Sum/1  "Clb"

== system VTOLDynamics/Force and Moments/Aerodynamic Forces/Compute Body Frame Forces and Moments/Wind frame F& M/Lateral Channel/Cn ==
  alpha : Inport
  beta : Inport  Port=2
  dA : Inport  Port=3
  dR : Inport  Port=4
  p,q,r : Inport  Port=5
  Airspeed : Inport  Port=6
  1-D Lookup Table : Lookup_n-D  BreakpointsForDimension1=uavParams.aero.alpha_latdir  BreakpointsForDimension2=uavParams.aero.beta_latdir  Table=uavParams.aero.CN  ExtrapMethod=Clip  UseLastTableValue=on  InternalRulePriority=Speed  RndMeth=Simplest
      settings: InputPortMap=u0,u1
  Abs : Abs  Commented=on  SaturateOnIntegerOverflow=off
  CnDa : Constant  Value=uavParams.aero.CnDa
      settings: AttributesFormatString=%<Value>
  CnDr : Constant  Value=uavParams.aero.CnDr
      settings: AttributesFormatString=%<Value>
  Cnb : Constant  Commented=on  Value=uavParam.aero.Cnb
      settings: AttributesFormatString=%<Value>
  Product1 : Product  SaturateOnIntegerOverflow=on  OutDataTypeStr=Inherit: Same as first input
  Product2 : Product  Commented=on
  Product5 : Product  SaturateOnIntegerOverflow=on  OutDataTypeStr=Inherit: Same as first input
  Sign : Signum  Commented=on
  Sum : Sum  Inputs=+++++  SaturateOnIntegerOverflow=on
  yaw factors : Subsystem
  Cn : Outport  VectorParamsAs1DForOutWhenUnconnected=off
  wires:
  Airspeed/1 -> yaw factors/2(Airspeed)
  p,q,r/1 -> yaw factors/1(p,q,r)
  CnDa/1 -> Product5/1
  Product5/1 -> Sum/2
  dA/1 -> Product5/2
  CnDr/1 -> Product1/1
  dR/1 -> Product1/2
  Sum/1 -> Cn/1
  Product1/1 -> Sum/3
  yaw factors/2(Cnr) -> Sum/5
  yaw factors/1(Cnp) -> Sum/4
  beta/1 -> 1-D Lookup Table/2
  alpha/1 -> 1-D Lookup Table/1
  1-D Lookup Table/1 -> Sum/1
  Sign/1 -> Product2/2

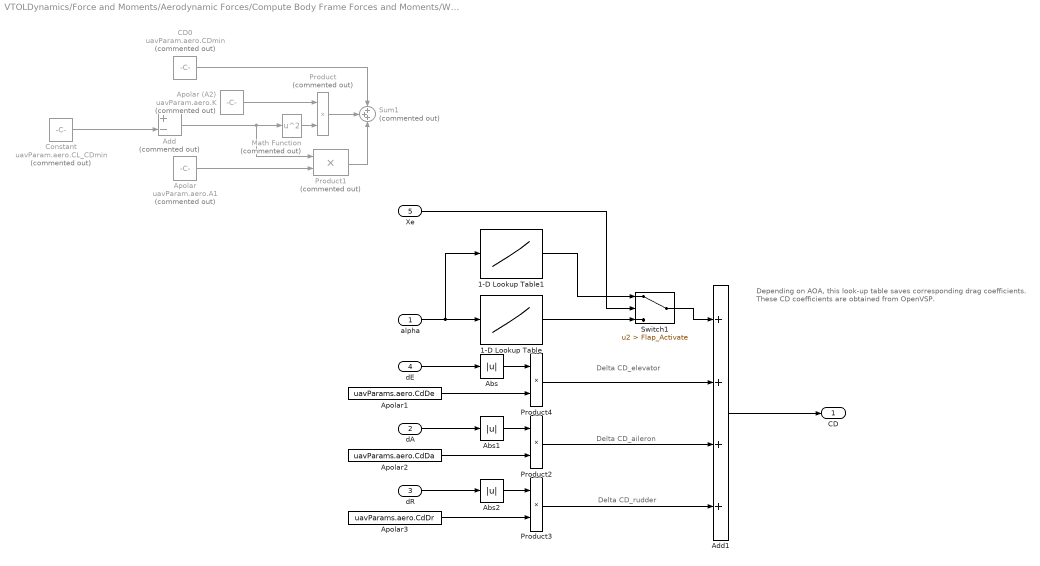
== system VTOLDynamics/Force and Moments/Aerodynamic Forces/Compute Body Frame Forces and Moments/Wind frame F& M/Longitudinal Channel/CD ==
  note: Delta CD_elevator
  note: Depending on AOA, this look-up table saves corresponding drag coefficients.
      | These CD coefficients are obtained from OpenVSP.
  note: Delta CD_aileron
  note: Delta CD_rudder
  alpha : Inport
  dA : Inport  Port=2
  dR : Inport  Port=3
  dE : Inport  Port=4
  Xe : Inport  Port=5
  1-D Lookup Table : Lookup_n-D  NumberOfTableDimensions=1  BreakpointsForDimension1=uavParams.aero.alpha_lon  Table=uavParams.aero.CD  ExtrapMethod=Clip  UseLastTableValue=on  InternalRulePriority=Speed  RndMeth=Simplest
  1-D Lookup Table1 : Lookup_n-D  NumberOfTableDimensions=1  BreakpointsForDimension1=uavParams.aero.alpha_lon  Table=uavParams.aero.CD_flap_20  ExtrapMethod=Clip  UseLastTableValue=on  InternalRulePriority=Speed  RndMeth=Simplest
  Abs : Abs  SaturateOnIntegerOverflow=off
  Abs1 : Abs  SaturateOnIntegerOverflow=off
  Abs2 : Abs  SaturateOnIntegerOverflow=off
  Add : Sum  Commented=on  Inputs=+-
  Add1 : Sum  Inputs=++++
  Apolar : Constant  Commented=on  Value=uavParam.aero.A1
      settings: AttributesFormatString=%<Value>
  Apolar (A2) : Constant  Commented=on  Value=uavParam.aero.K
      settings: AttributesFormatString=%<Value>
  Apolar1 : Constant  Value=uavParams.aero.CdDe
      settings: AttributesFormatString=%<Value>
  Apolar2 : Constant  Value=uavParams.aero.CdDa
      settings: AttributesFormatString=%<Value>
  Apolar3 : Constant  Value=uavParams.aero.CdDr
      settings: AttributesFormatString=%<Value>
  CD0 : Constant  Commented=on  Value=uavParam.aero.CDmin
      settings: AttributesFormatString=%<Value>
  Constant : Constant  Commented=on  Value=uavParam.aero.CL_CDmin
  Math Function : Math  Commented=on  Operator=square  SignedPower=on
  Product : Product  Commented=on  SaturateOnIntegerOverflow=on  OutDataTypeStr=Inherit: Same as first input
  Product1 : Product  Commented=on  SaturateOnIntegerOverflow=on  OutDataTypeStr=Inherit: Same as first input
  Product2 : Product  SaturateOnIntegerOverflow=on  OutDataTypeStr=Inherit: Same as first input
  Product3 : Product  SaturateOnIntegerOverflow=on  OutDataTypeStr=Inherit: Same as first input
  Product4 : Product  SaturateOnIntegerOverflow=on  OutDataTypeStr=Inherit: Same as first input
  Sum1 : Sum  Commented=on  Inputs=+++  SaturateOnIntegerOverflow=on
  Switch1 : Switch  Criteria=u2 > Threshold  Threshold=Flap_Activate  SaturateOnIntegerOverflow=off  InputSameDT=off
  CD : Outport  VectorParamsAs1DForOutWhenUnconnected=off
  wires:
  Add1/1 -> CD/1
  Apolar (A2)/1 -> Product/1
  Math Function/1 -> Product/2
  Product1/1 -> Sum1/3
  Product/1 -> Sum1/2
  Add/1 -> Product1/1, Math Function/1
  CD0/1 -> Sum1/1
  Apolar/1 -> Product1/2
  Constant/1 -> Add/2
  Apolar1/1 -> Product4/2
  dE/1 -> Abs/1
  Abs/1 -> Product4/1
  Abs1/1 -> Product2/1
  Apolar2/1 -> Product2/2
  dA/1 -> Abs1/1
  Abs2/1 -> Product3/1
  Apolar3/1 -> Product3/2
  dR/1 -> Abs2/1
  Product4/1 -> Add1/2
  Product2/1 -> Add1/3
  Product3/1 -> Add1/4
  Xe/1 -> Switch1/2
  alpha/1 -> 1-D Lookup Table1/1, 1-D Lookup Table/1
  1-D Lookup Table1/1 -> Switch1/1
  1-D Lookup Table/1 -> Switch1/3
  Switch1/1 -> Add1/1

== system VTOLDynamics/Force and Moments/Aerodynamic Forces/Compute Body Frame Forces and Moments/Wind frame F& M/Longitudinal Channel/CL ==
  alpha : Inport
  alpha_dot : Inport  Port=2
  dE : Inport  Port=3
  p,q,r : Inport  Port=4
  Airspeed : Inport  Port=5
  dA : Inport  Port=6
  Xe : Inport  Port=7
  1-D Lookup Table : Lookup_n-D  NumberOfTableDimensions=1  BreakpointsForDimension1=uavParams.aero.alpha_lon  Table=uavParams.aero.CL  ExtrapMethod=Clip  UseLastTableValue=on  InternalRulePriority=Speed  RndMeth=Simplest
  1-D Lookup Table1 : Lookup_n-D  NumberOfTableDimensions=1  BreakpointsForDimension1=uavParams.aero.alpha_lon  Table=uavParams.aero.CL_flap_20  ExtrapMethod=Clip  UseLastTableValue=on  InternalRulePriority=Speed  RndMeth=Simplest
  Abs : Abs  SaturateOnIntegerOverflow=off
  CL1 : Constant  Value=uavParams.aero.CLDa
      settings: AttributesFormatString=%<Value>
  CLDe : Constant  Value=uavParams.aero.CLDe
      settings: AttributesFormatString=%<Value>
  CLa_dot : Constant  Value=uavParams.aero.CLadot
      settings: AttributesFormatString=%<Value>
  Lift due to pitch rate : Subsystem
  Product1 : Product  SaturateOnIntegerOverflow=on  OutDataTypeStr=Inherit: Same as first input
  Product2 : Product  SaturateOnIntegerOverflow=on  OutDataTypeStr=Inherit: Same as first input
  Product5 : Product  SaturateOnIntegerOverflow=on  OutDataTypeStr=Inherit: Same as first input
  Sum : Sum  Inputs=+++++  SaturateOnIntegerOverflow=on
  Switch1 : Switch  Criteria=u2 > Threshold  Threshold=Flap_Activate  SaturateOnIntegerOverflow=off  InputSameDT=off
  CL : Outport  VectorParamsAs1DForOutWhenUnconnected=off
  wires:
  Airspeed/1 -> Lift due to pitch rate/2(Airspeed)
  p,q,r/1 -> Lift due to pitch rate/1(p,q,r)
  Sum/1 -> CL/1
  dE/1 -> Product1/2
  CLDe/1 -> Product1/1
  alpha_dot/1 -> Product5/2
  CLa_dot/1 -> Product5/1
  CL1/1 -> Product2/2
  dA/1 -> Abs/1
  Abs/1 -> Product2/1
  Product5/1 -> Sum/2
  Lift due to pitch rate/1(CLq) -> Sum/5
  Product1/1 -> Sum/3
  Product2/1 -> Sum/4
  alpha/1 -> 1-D Lookup Table/1, 1-D Lookup Table1/1
  Xe/1 -> Switch1/2
  1-D Lookup Table1/1 -> Switch1/1
  1-D Lookup Table/1 -> Switch1/3
  Switch1/1 -> Sum/1

== system VTOLDynamics/Force and Moments/Aerodynamic Forces/Compute Body Frame Forces and Moments/Wind frame F& M/Longitudinal Channel/Cm ==
  alpha : Inport
  dE : Inport  Port=2
  p,q,r : Inport  Port=3
  Airspeed : Inport  Port=4
  Xe : Inport  Port=5
  1-D Lookup Table : Lookup_n-D  NumberOfTableDimensions=1  BreakpointsForDimension1=uavParams.aero.alpha_lon  Table=uavParams.aero.CM  ExtrapMethod=Clip  UseLastTableValue=on  InternalRulePriority=Speed  RndMeth=Simplest
  1-D Lookup Table1 : Lookup_n-D  NumberOfTableDimensions=1  BreakpointsForDimension1=uavParams.aero.alpha_lon  Table=uavParams.aero.CM_flap_20  ExtrapMethod=Clip  UseLastTableValue=on  InternalRulePriority=Speed  RndMeth=Simplest
  CmDe : Constant  Value=uavParams.aero.CmDe
      settings: AttributesFormatString=%<Value>
  Lift due to pitch rate : Subsystem
  Product1 : Product  Inputs=**  SaturateOnIntegerOverflow=on  OutDataTypeStr=Inherit: Same as first input
  Sum : Sum  Inputs=+++  SaturateOnIntegerOverflow=on
  Switch1 : Switch  Criteria=u2 > Threshold  Threshold=Flap_Activate  SaturateOnIntegerOverflow=off  InputSameDT=off
  Cm : Outport  VectorParamsAs1DForOutWhenUnconnected=off
  wires:
  Lift due to pitch rate/1(Cmq) -> Sum/3  "cmq"
  p,q,r/1 -> Lift due to pitch rate/1(p,q,r)
  Sum/1 -> Cm/1  "total"
  dE/1 -> Product1/2
  CmDe/1 -> Product1/1
  Airspeed/1 -> Lift due to pitch rate/2(Airspeed)
  Product1/1 -> Sum/2  "cmde"
  Xe/1 -> Switch1/2
  alpha/1 -> 1-D Lookup Table/1, 1-D Lookup Table1/1
  1-D Lookup Table1/1 -> Switch1/1  "cma"
  1-D Lookup Table/1 -> Switch1/3  "cma"
  Switch1/1 -> Sum/1

== system VTOLDynamics/Force and Moments/Aerodynamic Forces/Compute Body Frame Forces and Moments/Wind frame F& M_original/Lateral Channel/CY ==
  beta : Inport
  dR : Inport  Port=2
  p,q,r : Inport  Port=3
  Airspeed : Inport  Port=4
  CYDr : Constant  Value=uavParam.aero.CYDr
      settings: AttributesFormatString=%<Value>
  CYb : Constant  Value=uavParam.aero.CYb
      settings: AttributesFormatString=%<Value>
  Gain : Gain  Gain=-1
  Product : Product  SaturateOnIntegerOverflow=on  OutDataTypeStr=Inherit: Same as first input
  Product1 : Product  SaturateOnIntegerOverflow=on  OutDataTypeStr=Inherit: Same as first input
  Sum2 : Sum  Inputs=++++  SaturateOnIntegerOverflow=on
  roll factors : Subsystem
  CY : Outport  VectorParamsAs1DForOutWhenUnconnected=off
  wires:
  Product1/1 -> Sum2/2
  dR/1 -> Product1/2
  CYDr/1 -> Product1/1
  Product/1 -> Sum2/1
  beta/1 -> Product/2
  CYb/1 -> Product/1
  Sum2/1 -> Gain/1
  Airspeed/1 -> roll factors/2(Airspeed)
  p,q,r/1 -> roll factors/1(p,q,r)
  roll factors/1(CYp) -> Sum2/3
  roll factors/2(CYr) -> Sum2/4
  Gain/1 -> CY/1

== system VTOLDynamics/Force and Moments/Aerodynamic Forces/Compute Body Frame Forces and Moments/Wind frame F& M_original/Lateral Channel/Cl ==
  beta : Inport
  dA : Inport  Port=2
  dR : Inport  Port=3
  p,q,r : Inport  Port=4
  Airspeed : Inport  Port=5
  ClDa : Constant  Value=uavParam.aero.ClDa
      settings: AttributesFormatString=%<Value>
  ClDr : Constant  Value=uavParam.aero.ClDr
      settings: AttributesFormatString=%<Value>
  Clb : Constant  Value=uavParam.aero.Clb
      settings: AttributesFormatString=%<Value>
  Product1 : Product  SaturateOnIntegerOverflow=on  OutDataTypeStr=Inherit: Same as first input
  Product4 : Product  SaturateOnIntegerOverflow=on  OutDataTypeStr=Inherit: Same as first input
  Product5 : Product  SaturateOnIntegerOverflow=on  OutDataTypeStr=Inherit: Same as first input
  Sum : Sum  Inputs=+++++  SaturateOnIntegerOverflow=on
  roll factors : Subsystem
  Cl : Outport  VectorParamsAs1DForOutWhenUnconnected=off
  wires:
  roll factors/1(Clp) -> Sum/4
  Product5/1 -> Sum/2  "CldA"
  Airspeed/1 -> roll factors/2(Airspeed)
  p,q,r/1 -> roll factors/1(p,q,r)
  roll factors/2(Clr) -> Sum/5
  Product1/1 -> Sum/3  "Cldr"
  Product4/1 -> Sum/1  "Clb"
  Sum/1 -> Cl/1
  dR/1 -> Product1/2
  ClDr/1 -> Product1/1
  dA/1 -> Product5/2
  ClDa/1 -> Product5/1
  beta/1 -> Product4/2
  Clb/1 -> Product4/1

== system VTOLDynamics/Force and Moments/Aerodynamic Forces/Compute Body Frame Forces and Moments/Wind frame F& M_original/Lateral Channel/Cn ==
  beta : Inport
  dA : Inport  Port=2
  dR : Inport  Port=3
  p,q,r : Inport  Port=4
  Airspeed : Inport  Port=5
  CnDa : Constant  Value=uavParam.aero.CnDa
      settings: AttributesFormatString=%<Value>
  CnDr : Constant  Value=uavParam.aero.CnDr
      settings: AttributesFormatString=%<Value>
  Cnb : Constant  Value=uavParam.aero.Cnb
      settings: AttributesFormatString=%<Value>
  Product1 : Product  SaturateOnIntegerOverflow=on  OutDataTypeStr=Inherit: Same as first input
  Product4 : Product  SaturateOnIntegerOverflow=on  OutDataTypeStr=Inherit: Same as first input
  Product5 : Product  SaturateOnIntegerOverflow=on  OutDataTypeStr=Inherit: Same as first input
  Sum : Sum  Inputs=+++++  SaturateOnIntegerOverflow=on
  yaw factors : Subsystem
  Cn : Outport  VectorParamsAs1DForOutWhenUnconnected=off
  wires:
  Airspeed/1 -> yaw factors/2(Airspeed)
  p,q,r/1 -> yaw factors/1(p,q,r)
  Cnb/1 -> Product4/1
  beta/1 -> Product4/2
  CnDa/1 -> Product5/1
  Product5/1 -> Sum/2
  dA/1 -> Product5/2
  CnDr/1 -> Product1/1
  dR/1 -> Product1/2
  Sum/1 -> Cn/1
  Product1/1 -> Sum/3
  yaw factors/2(Cnr) -> Sum/5
  yaw factors/1(Cnp) -> Sum/4
  Product4/1 -> Sum/1

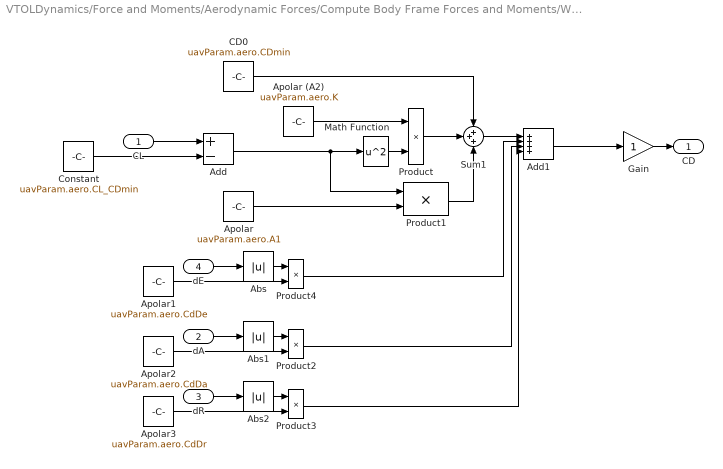
== system VTOLDynamics/Force and Moments/Aerodynamic Forces/Compute Body Frame Forces and Moments/Wind frame F& M_original/Longitudinal Channel/CD ==
  CL : Inport
  dA : Inport  Port=2
  dR : Inport  Port=3
  dE : Inport  Port=4
  Abs : Abs  SaturateOnIntegerOverflow=off
  Abs1 : Abs  SaturateOnIntegerOverflow=off
  Abs2 : Abs  SaturateOnIntegerOverflow=off
  Add : Sum  Inputs=+-
  Add1 : Sum  Inputs=++++
  Apolar : Constant  Value=uavParam.aero.A1
      settings: AttributesFormatString=%<Value>
  Apolar (A2) : Constant  Value=uavParam.aero.K
      settings: AttributesFormatString=%<Value>
  Apolar1 : Constant  Value=uavParam.aero.CdDe
      settings: AttributesFormatString=%<Value>
  Apolar2 : Constant  Value=uavParam.aero.CdDa
      settings: AttributesFormatString=%<Value>
  Apolar3 : Constant  Value=uavParam.aero.CdDr
      settings: AttributesFormatString=%<Value>
  CD0 : Constant  Value=uavParam.aero.CDmin
      settings: AttributesFormatString=%<Value>
  Constant : Constant  Value=uavParam.aero.CL_CDmin
  Gain : Gain  SaturateOnIntegerOverflow=on  OutDataTypeStr=Inherit: Same as input  ParamDataTypeStr=Inherit: Same as input
      settings: AttributesFormatString=%<Gain>
  Math Function : Math  Operator=square  SignedPower=on
  Product{,1..4} (5 alike) : Product  SaturateOnIntegerOverflow=on  OutDataTypeStr=Inherit: Same as first input
  Sum1 : Sum  Inputs=+++  SaturateOnIntegerOverflow=on
  CD : Outport  VectorParamsAs1DForOutWhenUnconnected=off
  wires:
  Gain/1 -> CD/1
  Apolar (A2)/1 -> Product/1
  Math Function/1 -> Product/2
  Product1/1 -> Sum1/3
  Product/1 -> Sum1/2
  Add/1 -> Product1/1, Math Function/1
  CD0/1 -> Sum1/1
  Apolar/1 -> Product1/2
  CL/1 -> Add/1
  Constant/1 -> Add/2
  Apolar1/1 -> Product4/2
  dE/1 -> Abs/1
  Abs/1 -> Product4/1
  Abs1/1 -> Product2/1
  Apolar2/1 -> Product2/2
  dA/1 -> Abs1/1
  Abs2/1 -> Product3/1
  Apolar3/1 -> Product3/2
  dR/1 -> Abs2/1
  Sum1/1 -> Add1/1
  Add1/1 -> Gain/1
  Product4/1 -> Add1/2
  Product2/1 -> Add1/3
  Product3/1 -> Add1/4

== system VTOLDynamics/Force and Moments/Aerodynamic Forces/Compute Body Frame Forces and Moments/Wind frame F& M_original/Longitudinal Channel/CL ==
  alpha : Inport
  alpha_dot : Inport  Port=2
  dE : Inport  Port=3
  p,q,r : Inport  Port=4
  Airspeed : Inport  Port=5
  dA : Inport  Port=6
  Abs : Abs  SaturateOnIntegerOverflow=off
  CL0 : Constant  Value=uavParam.aero.CL0
      settings: AttributesFormatString=%<Value>
  CL1 : Constant  Value=uavParam.aero.CLDa
      settings: AttributesFormatString=%<Value>
  CLDe : Constant  Value=uavParam.aero.CLDe
      settings: AttributesFormatString=%<Value>
  CLa : Constant  Value=uavParam.aero.CLa
      settings: AttributesFormatString=%<Value>
  CLa_dot : Constant  Value=uavParam.aero.CLa_dot
      settings: AttributesFormatString=%<Value>
  Lift due to pitch rate : Subsystem
  Product{1..2,4..5} (4 alike) : Product  SaturateOnIntegerOverflow=on  OutDataTypeStr=Inherit: Same as first input
  Sum : Sum  Inputs=++++++  SaturateOnIntegerOverflow=on
  CL : Outport  VectorParamsAs1DForOutWhenUnconnected=off
  wires:
  CL0/1 -> Sum/1
  Airspeed/1 -> Lift due to pitch rate/2(Airspeed)
  p,q,r/1 -> Lift due to pitch rate/1(p,q,r)
  Product1/1 -> Sum/4
  Product5/1 -> Sum/3
  Sum/1 -> CL/1
  dE/1 -> Product1/2
  CLDe/1 -> Product1/1
  alpha_dot/1 -> Product5/2
  CLa_dot/1 -> Product5/1
  alpha/1 -> Product4/2
  CLa/1 -> Product4/1
  Product4/1 -> Sum/2
  Lift due to pitch rate/1(CLq) -> Sum/6
  CL1/1 -> Product2/2
  Product2/1 -> Sum/5
  dA/1 -> Abs/1
  Abs/1 -> Product2/1

== system VTOLDynamics/Force and Moments/Aerodynamic Forces/Compute Body Frame Forces and Moments/Wind frame F& M_original/Longitudinal Channel/Cm ==
  alpha : Inport
  De : Inport  Port=2
  p,q,r : Inport  Port=3
  Airspeed : Inport  Port=4
  Cm0 : Constant  Value=uavParam.aero.Cm0
      settings: AttributesFormatString=%<Value>
  CmDe : Constant  Value=uavParam.aero.CmDe
      settings: AttributesFormatString=%<Value>
  Cma : Constant  Value=uavParam.aero.Cma
      settings: AttributesFormatString=%<Value>
  Lift due to pitch rate : Subsystem
  Product1 : Product  Inputs=**  SaturateOnIntegerOverflow=on  OutDataTypeStr=Inherit: Same as first input
  Product4 : Product  SaturateOnIntegerOverflow=on  OutDataTypeStr=Inherit: Same as first input
  Sum : Sum  Inputs=+++++  SaturateOnIntegerOverflow=on
  Cm : Outport  VectorParamsAs1DForOutWhenUnconnected=off
  wires:
  Lift due to pitch rate/1(Cmq) -> Sum/5  "cmq"
  p,q,r/1 -> Lift due to pitch rate/1(p,q,r)
  Product1/1 -> Sum/3  "cmde"
  Product4/1 -> Sum/2  "cma"
  Sum/1 -> Cm/1  "total"
  De/1 -> Product1/2
  CmDe/1 -> Product1/1
  Cma/1 -> Product4/1
  Cm0/1 -> Sum/1  "cm0"
  Airspeed/1 -> Lift due to pitch rate/2(Airspeed)
  alpha/1 -> Product4/2
